simulink model "Motores_sensores"  (R2023b)
settings: Solver=VariableStepAuto  StartTime=0.0  StopTime=10.0  RelTol=1e-3
libraries: arduinolib x11, simulink x9
settings Model: Creator=andre  LastModifiedBy=pcele

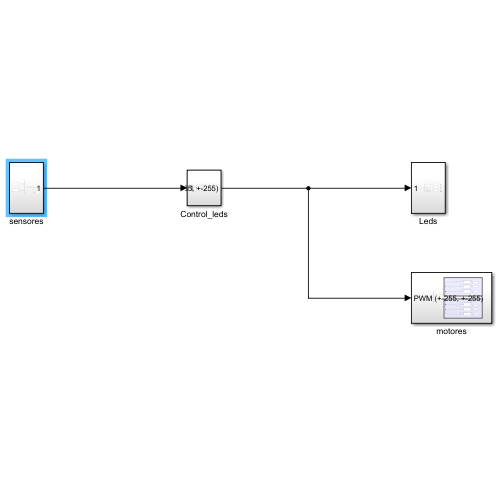
[thumbnail: Simulink's stored preview of the top-level diagram]
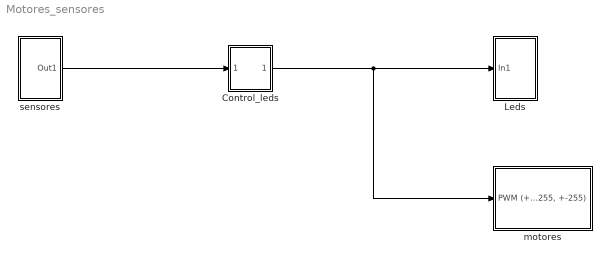
== system Motores_sensores ==
  Control_leds : Subsystem
  Leds : Subsystem
  motores : Subsystem
  sensores : Subsystem
  wires:
  sensores/1(Out1) -> Control_leds/1(In1)
  Control_leds/1("PWM (+-255, +-255)") -> motores/1("PWM (+-255, +-255)"), Leds/1(In1)

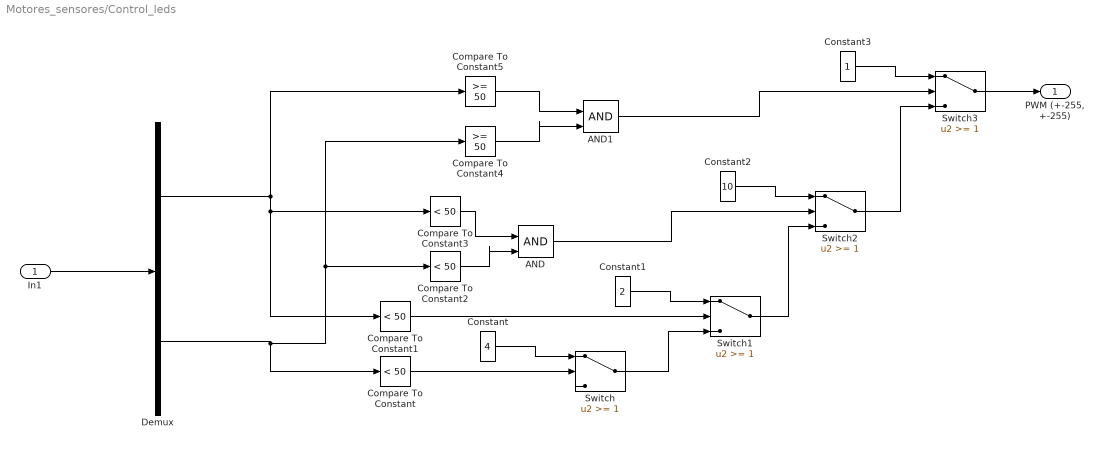
== system Motores_sensores/Control_leds ==
  In1 : Inport
  AND : Logic  IconShape=distinctive  AllPortsSameDT=off  OutDataTypeStr=boolean
  AND1 : Logic  IconShape=distinctive  AllPortsSameDT=off  OutDataTypeStr=boolean
  Compare To Constant{,1..3} (4 alike) : simulink/Logic and Bit Operations/Compare To Constant  relop=<  const=50  OutDataTypeStr=boolean
  Compare To Constant4 : simulink/Logic and Bit Operations/Compare To Constant  relop=>=  const=50  OutDataTypeStr=boolean
  Compare To Constant5 : simulink/Logic and Bit Operations/Compare To Constant  relop=>=  const=50  OutDataTypeStr=boolean
  Constant : Constant  Value=4  SampleTime=-1
  Constant1 : Constant  Value=2  SampleTime=-1
  Constant2 : Constant  Value=10  SampleTime=-1
  Constant3 : Constant  SampleTime=-1
  Demux : Demux  Outputs=2
  Switch{,1..3} (4 alike) : Switch  Threshold=1  SaturateOnIntegerOverflow=off  InputSameDT=off
  "PWM (+-255, +-255)" : Outport
  wires:
  Switch2/1 -> Switch3/3
  In1/1 -> Demux/1
  Compare To Constant2/1 -> AND/2
  Compare To Constant4/1 -> AND1/2
  Constant2/1 -> Switch2/1
  Demux/2 -> Compare To Constant4/1, Compare To Constant2/1, Compare To Constant/1
  Demux/1 -> Compare To Constant5/1, Compare To Constant1/1, Compare To Constant3/1
  Compare To Constant/1 -> Switch/2
  Switch3/1 -> "PWM (+-255, +-255)"/1
  Compare To Constant5/1 -> AND1/1
  Switch1/1 -> Switch2/3
  Constant/1 -> Switch/1
  Switch/1 -> Switch1/3
  Constant3/1 -> Switch3/1
  AND/1 -> Switch2/2
  AND1/1 -> Switch3/2
  Compare To Constant1/1 -> Switch1/2
  Compare To Constant3/1 -> AND/1
  Constant1/1 -> Switch1/1

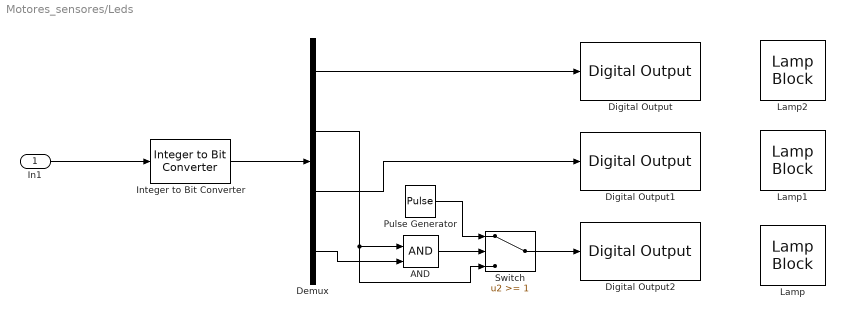
== system Motores_sensores/Leds ==
  In1 : Inport
  AND : Logic  IconShape=distinctive  AllPortsSameDT=off  OutDataTypeStr=boolean
  Demux : Demux
  Digital Output : arduinolib/Digital Output  pinNumber=49  Direction=output  blockPlatform=arduino
  Digital Output1 : arduinolib/Digital Output  pinNumber=51  Direction=output  blockPlatform=arduino
  Digital Output2 : arduinolib/Digital Output  pinNumber=53  Direction=output  blockPlatform=arduino
  Integer to Bit Converter : simulink/Logic and Bit Operations/Integer to Bit Converter  nbits=3  signedInputValues=Unsigned  bitOrder=LSB first  outDtype=boolean
  Lamp : LampBlock  LabelPosition=Hide
  Lamp1 : LampBlock  LabelPosition=Hide
  Lamp2 : LampBlock  LabelPosition=Hide
  Pulse Generator : DiscretePulseGenerator  PulseType=Time based  Period=10  PulseWidth=5
  Switch : Switch  Threshold=1  SaturateOnIntegerOverflow=off  InputSameDT=off
  wires:
  AND/1 -> Switch/2
  Demux/2 -> Switch/3, AND/1
  Demux/1 -> Digital Output/1
  In1/1 -> Integer to Bit Converter/1
  Demux/4 -> AND/2
  Switch/1 -> Digital Output2/1
  Demux/3 -> Digital Output1/1
  Pulse Generator/1 -> Switch/1
  Integer to Bit Converter/1 -> Demux/1

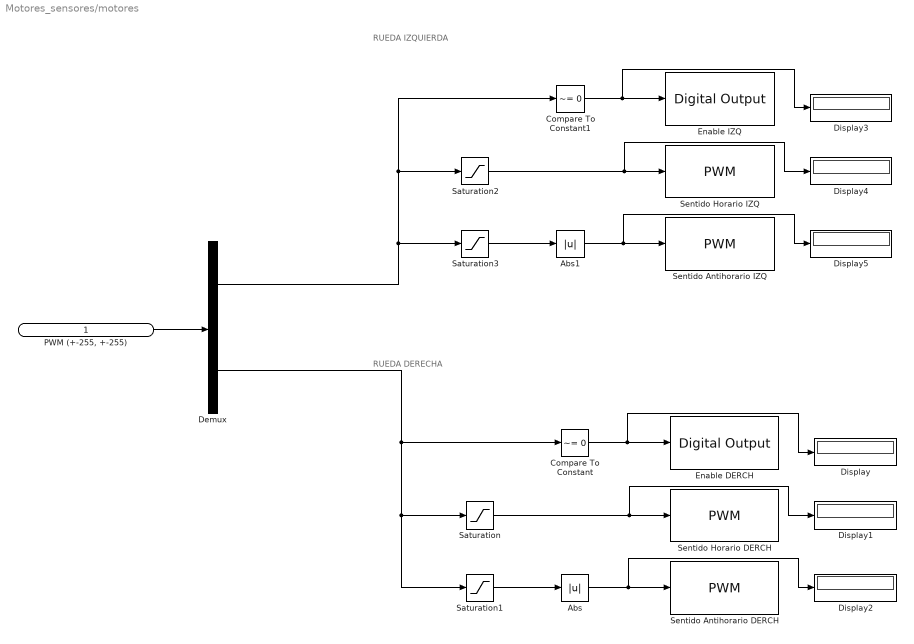
== system Motores_sensores/motores ==
  note: RUEDA IZQUIERDA
  note: RUEDA DERECHA
  "PWM (+-255, +-255)" : Inport
  Abs : Abs  SaturateOnIntegerOverflow=off
  Abs1 : Abs  SaturateOnIntegerOverflow=off
  Compare To Constant : simulink/Logic and Bit Operations/Compare To Constant  relop=~=  const=0  OutDataTypeStr=boolean
  Compare To Constant1 : simulink/Logic and Bit Operations/Compare To Constant  relop=~=  const=0  OutDataTypeStr=boolean
  Demux : Demux  Outputs=2
  Display{,1..5} (6 alike) : Display
  Enable DERCH : arduinolib/Digital Output  pinNumber=13  Direction=output  blockPlatform=arduino
  Enable IZQ : arduinolib/Digital Output  pinNumber=8  Direction=output  blockPlatform=arduino
  Saturation : Saturate  UpperLimit=255  LowerLimit=0
  Saturation1 : Saturate  UpperLimit=0  LowerLimit=-255
  Saturation2 : Saturate  UpperLimit=255  LowerLimit=0
  Saturation3 : Saturate  UpperLimit=0  LowerLimit=-255
  Sentido Antihorario DERCH : arduinolib/PWM  pinNumber=12  frequencyType=Default  desiredFrequency=490.2  achievableFrequency=490.2
  Sentido Antihorario IZQ : arduinolib/PWM  pinNumber=10  frequencyType=Default  desiredFrequency=490.2  achievableFrequency=490.2
  Sentido Horario DERCH : arduinolib/PWM  pinNumber=11  frequencyType=Default  desiredFrequency=490.2  achievableFrequency=490.2
  Sentido Horario IZQ : arduinolib/PWM  pinNumber=9  frequencyType=Default  desiredFrequency=490.2  achievableFrequency=490.2
  wires:
  Saturation3/1 -> Abs1/1
  Abs/1 -> Display2/1, Sentido Antihorario DERCH/1
  Demux/2 -> Saturation1/1, Saturation/1, Compare To Constant/1
  Abs1/1 -> Display5/1, Sentido Antihorario IZQ/1
  Compare To Constant1/1 -> Display3/1, Enable IZQ/1
  Demux/1 -> Compare To Constant1/1, Saturation2/1, Saturation3/1
  Saturation2/1 -> Sentido Horario IZQ/1, Display4/1
  Saturation/1 -> Sentido Horario DERCH/1, Display1/1
  Compare To Constant/1 -> Display/1, Enable DERCH/1
  Saturation1/1 -> Abs/1
  "PWM (+-255, +-255)"/1 -> Demux/1

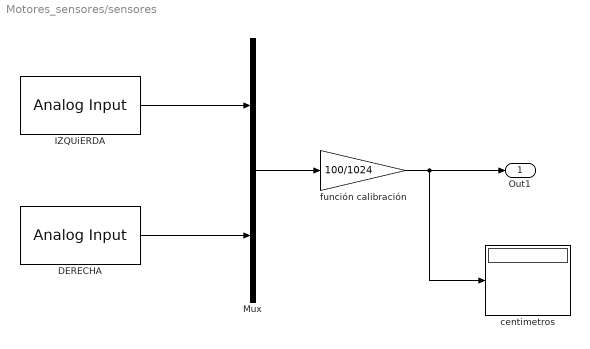
== system Motores_sensores/sensores ==
  DERECHA : arduinolib/Analog Input  pinNumber=3  ReadResultsOnly=off  ConversionTriggerSource=Software  ExternalTriggerType=uint32( 0 )  OutputDataType=uint16  EnableConversionCompleteNotify=off  EnableOuputStatus=off  SampleTime=-1  blockPlatform=arduino
  IZQUiERDA : arduinolib/Analog Input  pinNumber=7  ReadResultsOnly=off  ConversionTriggerSource=Software  ExternalTriggerType=uint32( 0 )  OutputDataType=uint16  EnableConversionCompleteNotify=off  EnableOuputStatus=off  SampleTime=-1  blockPlatform=arduino
  Mux : Mux  Inputs=2
  centimetros : Display
  función calibración : Gain  Gain=100/1024
  Out1 : Outport
  wires:
  DERECHA/1 -> Mux/2
  función calibración/1 -> centimetros/1, Out1/1
  Mux/1 -> función calibración/1
  IZQUiERDA/1 -> Mux/1
